simulink model "SmoothTrajFilters"  (R2017b)
settings: Solver=ode4  StartTime=0.0  StopTime=20  FixedStep=sim_step  RelTol=1e-3  EnableMultiTasking=on
settings Model: Creator=Burak  LastModifiedBy=buyue
settings DataIOCC: LimitDataPoints=on  SaveFormat=Array
settings OptimizationCC: LifeSpan=inf
settings DebuggingCC: UnderspecifiedInitializationDetection=Classic  MergeDetectMultiDrivingBlocksExec=none  SolverPrmCheckMsg=warning  StateNameClashWarn=warning  SFUnexpectedBacktrackingDiag=warning  SFNoUnconditionalDefaultTransitionDiag=warning  SFExecutionAtInitializationDiag=none
settings HardwareCC: ProdBitPerPointer=32  ProdBitPerSizeT=32  ProdBitPerPtrDiffT=32  ProdLargestAtomicFloat=None  ProdIntDivRoundTo=Undefined  ProdEndianess=Unspecified  ProdWordSize=32  ProdHWDeviceType=32-bit Generic
settings ModelReferenceCC: PropagateSignalLabelsOutOfModel=off
settings CodeAppCC: StateflowObjectComments=on
settings GRTTargetCC: TargetLangStandard=C89/C90 (ANSI)  GeneratePreprocessorConditionals=Disable all
settings ConfigComp: CovMetricSettings=dw  CovHtmlReporting=on  CovSaveCumulativeToWorkspaceVar=on  CovSaveSingleToWorkspaceVar=on  CovExternalEMLEnable=off

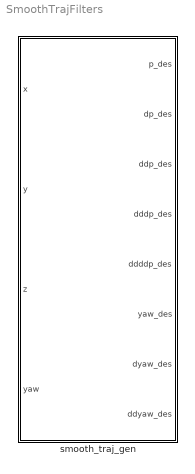
== system SmoothTrajFilters ==
  smooth_traj_gen : Subsystem  Description=|
      | % LTI-second and fourth order.
      | % Second and Fourth order smooth differentiator
      | % From 3D position and 1D yaw set points
      | % Code part of Lecture IAR @IST-Uni Stuttgart
      | % Author: Burak Yueksel

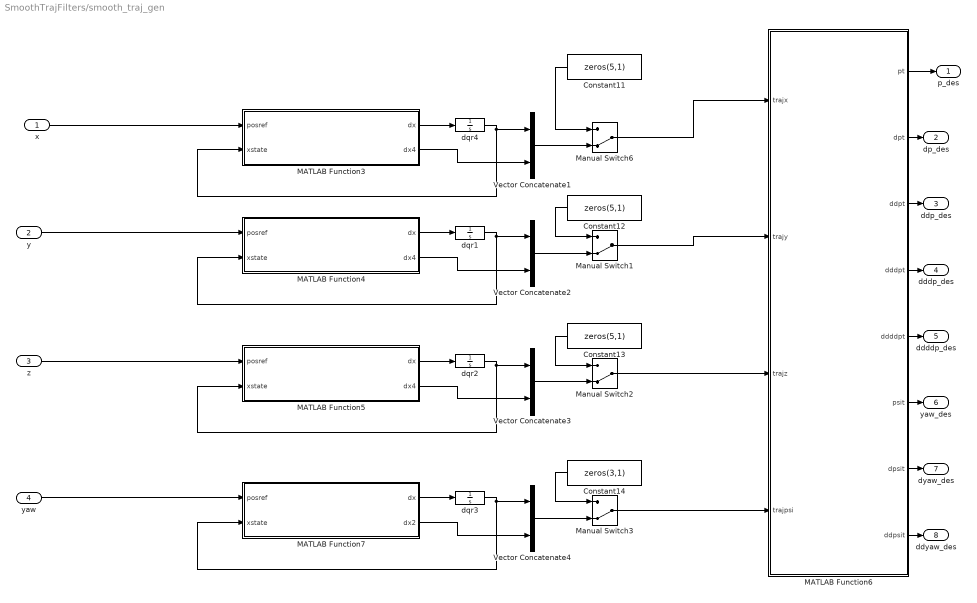
== system SmoothTrajFilters/smooth_traj_gen ==
  x : Inport
  y : Inport  Port=2
  z : Inport  Port=3
  yaw : Inport  Port=4
  Constant11 : Constant  Value=zeros(5,1)
  Constant12 : Constant  Value=zeros(5,1)
  Constant13 : Constant  Value=zeros(5,1)
  Constant14 : Constant  Value=zeros(3,1)
  MATLAB Function3 : MATLAB Function  Description=|  TreatAsAtomicUnit=on
      | % LTI fourth order.
      | % Fourth order smooth differentiator
      | % From 3D position set points
      | % Code part of Lecture IAR @IST-Uni Stuttgart
      | % Author: Burak Yueksel
  MATLAB Function4 : MATLAB Function  Description=|  TreatAsAtomicUnit=on
      | % LTI fourth order.
      | % Fourth order smooth differentiator
      | % From 3D position set points
      | % Code part of Lecture IAR @IST-Uni Stuttgart
      | % Author: Burak Yueksel
  MATLAB Function5 : MATLAB Function  Description=|  TreatAsAtomicUnit=on
      | % LTI fourth order.
      | % Fourth order smooth differentiator
      | % From 3D position set points
      | % Code part of Lecture IAR @IST-Uni Stuttgart
      | % Author: Burak Yueksel
  MATLAB Function6 : MATLAB Function  TreatAsAtomicUnit=on
  MATLAB Function7 : MATLAB Function  Description=|  TreatAsAtomicUnit=on
      | % LTI second order.
      | % Second order smooth differentiator
      | % From 1D yaw set points
      | % Code part of Lecture IAR @IST-Uni Stuttgart
      | % Author: Burak Yueksel
  Manual Switch{1..3,6} (4 alike) : ManualSwitch  CurrentSetting=0
  Vector Concatenate{1..4} (4 alike) : Concatenate
  dqr1 : Integrator  InitialCondition=[0,0,0,0];
  dqr2 : Integrator  InitialCondition=[0,0,0,0];
  dqr3 : Integrator  InitialCondition=[0,0];
  dqr4 : Integrator  InitialCondition=[0,0,0,0];
  p_des : Outport
  dp_des : Outport  Port=2
  ddp_des : Outport  Port=3
  dddp_des : Outport  Port=4
  ddddp_des : Outport  Port=5
  yaw_des : Outport  Port=6
  dyaw_des : Outport  Port=7
  ddyaw_des : Outport  Port=8
  wires:
  MATLAB Function6/1(pt) -> p_des/1
  MATLAB Function7/2(dx2) -> Vector Concatenate4/2
  x/1 -> MATLAB Function3/1(posref)
  dqr2/1 -> Vector Concatenate3/1, MATLAB Function5/2(xstate)
  MATLAB Function3/1(dx) -> dqr4/1
  MATLAB Function7/1(dx) -> dqr3/1
  yaw/1 -> MATLAB Function7/1(posref)
  MATLAB Function5/2(dx4) -> Vector Concatenate3/2
  Constant14/1 -> Manual Switch3/1
  Manual Switch3/1 -> MATLAB Function6/4(trajpsi)
  MATLAB Function4/1(dx) -> dqr1/1
  MATLAB Function3/2(dx4) -> Vector Concatenate1/2
  MATLAB Function5/1(dx) -> dqr2/1
  Constant13/1 -> Manual Switch2/1
  MATLAB Function4/2(dx4) -> Vector Concatenate2/2
  Vector Concatenate2/1 -> Manual Switch1/2
  Vector Concatenate1/1 -> Manual Switch6/2
  Constant11/1 -> Manual Switch6/1
  Vector Concatenate3/1 -> Manual Switch2/2
  Manual Switch6/1 -> MATLAB Function6/1(trajx)
  Constant12/1 -> Manual Switch1/1
  Manual Switch1/1 -> MATLAB Function6/2(trajy)
  y/1 -> MATLAB Function4/1(posref)
  z/1 -> MATLAB Function5/1(posref)
  dqr3/1 -> Vector Concatenate4/1, MATLAB Function7/2(xstate)
  dqr4/1 -> Vector Concatenate1/1, MATLAB Function3/2(xstate)
  dqr1/1 -> Vector Concatenate2/1, MATLAB Function4/2(xstate)
  Vector Concatenate4/1 -> Manual Switch3/2
  Manual Switch2/1 -> MATLAB Function6/3(trajz)
  MATLAB Function6/4(dddpt) -> dddp_des/1
  MATLAB Function6/2(dpt) -> dp_des/1
  MATLAB Function6/5(ddddpt) -> ddddp_des/1
  MATLAB Function6/6(psit) -> yaw_des/1
  MATLAB Function6/8(ddpsit) -> ddyaw_des/1
  MATLAB Function6/7(dpsit) -> dyaw_des/1
  MATLAB Function6/3(ddpt) -> ddp_des/1

== matlab function SmoothTrajFilters/smooth_traj_gen/MATLAB Function4 ==
  data: posref input; dx output; xstate input; K_trajy parameter; dx4 output
function [dx,dx4]  = trajectory(posref,xstate,K_trajy)
% LTI-fourth order.
% Fourth order smooth differentiator
% Code part of Lecture IAR @IST-Uni Stuttgart
% Author: Burak Yueksel
A=[0 1 0 0; 0 0 1 0; 0 0 0 1; 0 0 0 0];
B=[0 0 0 1]';
dx=(A-B*K_trajy)*(xstate-[posref;0;0;0]);
dx4=dx(4);
end

== matlab function SmoothTrajFilters/smooth_traj_gen/MATLAB Function3 ==
  data: posref input; dx output; xstate input; K_trajx parameter; dx4 output
function [dx,dx4]  = trajectory(posref,xstate,K_trajx)
% LTI-fourth order.
% Fourth order smooth differentiator
% Code part of Lecture IAR @IST-Uni Stuttgart
% Author: Burak Yueksel
A=[0 1 0 0; 0 0 1 0; 0 0 0 1; 0 0 0 0];
B=[0 0 0 1]';
dx=(A-B*K_trajx)*(xstate-[posref;0;0;0]);
dx4=dx(4);
end

== matlab function SmoothTrajFilters/smooth_traj_gen/MATLAB Function5 ==
  data: posref input; dx output; xstate input; K_trajz parameter; dx4 output
function [dx,dx4]  = trajectory(posref,xstate,K_trajz)
% LTI-fourth order.
% Fourth order smooth differentiator
% Code part of Lecture IAR @IST-Uni Stuttgart
% Author: Burak Yueksel
A=[0 1 0 0; 0 0 1 0; 0 0 0 1; 0 0 0 0];
B=[0 0 0 1]';
dx=(A-B*K_trajz)*(xstate-[posref;0;0;0]);
dx4=dx(4);
end

== matlab function SmoothTrajFilters/smooth_traj_gen/MATLAB Function6 ==
  data: pt output; dpt output; ddpt output; dddpt output; ddddpt output; trajx input; trajy input; trajz input; trajpsi input; psit output; dpsit output; ddpsit output
function [pt, dpt, ddpt, dddpt, ddddpt, psit, dpsit, ddpsit] = trajgen(trajx,trajy,trajz,trajpsi)
% simple i/o block
pt=zeros(3,1);
dpt=zeros(3,1);
ddpt=zeros(3,1);
dddpt=zeros(3,1);
ddddpt=zeros(3,1);
pt(1) = trajx(1);
pt(2) = trajy(1);
pt(3) = trajz(1);
dpt(1) = trajx(2);
dpt(2) = trajy(2);
dpt(3) = trajz(2);
ddpt(1) = trajx(3);
ddpt(2) = trajy(3);
ddpt(3) = trajz(3);
dddpt(1) = trajx(4);
dddpt(2) = trajy(4);
dddpt(3) = trajz(4);
ddddpt(1) = trajx(5);
ddddpt(2) = trajy(5);
ddddpt(3) = trajz(5);
psit = trajpsi(1);
dpsit = trajpsi(2);
ddpsit = trajpsi(3);

== matlab function SmoothTrajFilters/smooth_traj_gen/MATLAB Function7 ==
  data: posref input; dx output; xstate input; K_trajpsi parameter; dx2 output
function [dx,dx2]  = trajectory(posref,xstate,K_trajpsi)
% LTI-second order.
% Second order smooth differentiator
% Code part of Lecture IAR @IST-Uni Stuttgart
% Author: Burak Yueksel
A=[0 1 ; 0 0];
B=[0 1]';
dx=(A-B*K_trajpsi)*(xstate-[posref;0]);
dx2=dx(2);
end
